simulink model "ForTest"  (R2023a)
settings: configuration reference "Reference" (kept outside this file)
libraries: trse_cmn_lib_V2 x2
settings Model: DataDictionary=For_common_config.sldd  Creator=C3020  LastModifiedBy=C9166
settings ConfigSetRef: SourceName=Reference

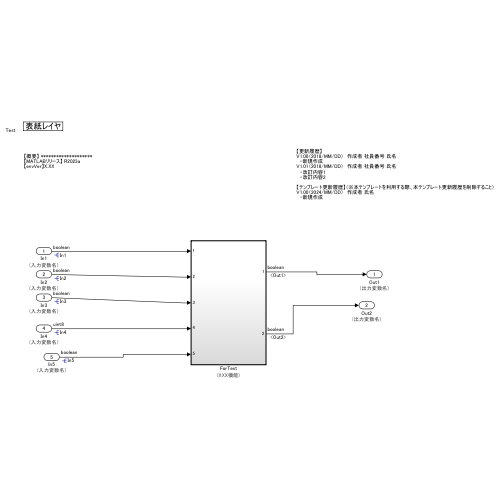
[thumbnail: Simulink's stored preview of the top-level diagram]
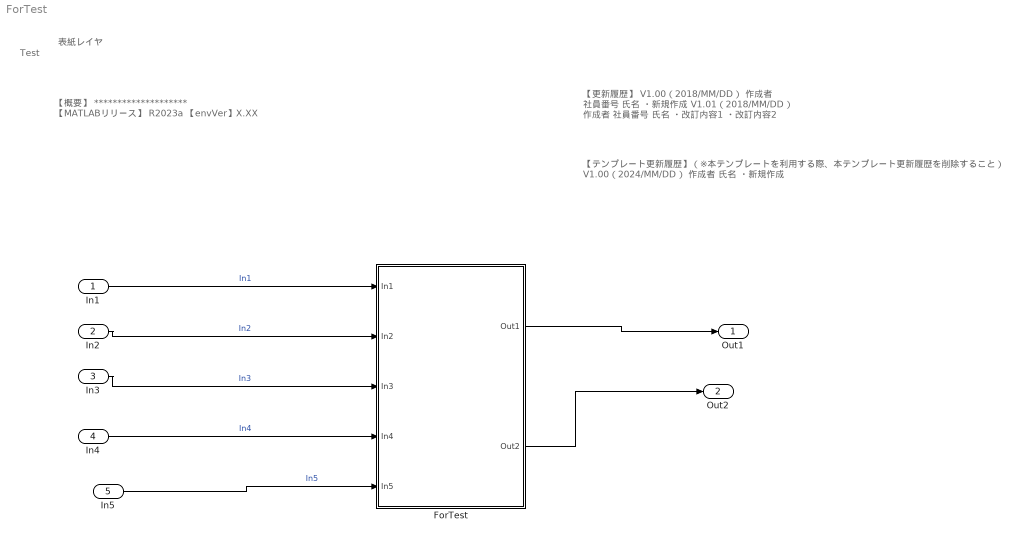
== system ForTest ==
  note: 表紙レイヤ
  note: 【更新履歴】
      | V1.00（2018/MM/DD）　作成者 社員番号 氏名
      | 　・新規作成
      | V1.01（2018/MM/DD）　作成者 社員番号 氏名
      | 　・改訂内容1
      | 　・改訂内容2
  note: 【テンプレート更新履歴】（※本テンプレートを利用する際、本テンプレート更新履歴を削除すること）
      | V1.00（2024/MM/DD）　作成者 氏名
      | 　・新規作成
  note: 【概要】 ********************
      | 【MATLABリリース】 R2023a
      | 【envVer】X.XX
  note: Test
  In1 : Inport  Description=入力変数名
      settings: AttributesFormatString=(%<Description>)
  In2 : Inport  Description=入力変数名  Port=2
      settings: AttributesFormatString=(%<Description>)
  In3 : Inport  Description=入力変数名  Port=3
      settings: AttributesFormatString=(%<Description>)
  In4 : Inport  Description=入力変数名  Port=4
      settings: AttributesFormatString=(%<Description>)
  In5 : Inport  Description=入力変数名  Port=5
      settings: AttributesFormatString=(%<Description>)
  ForTest : Subsystem  Description=XXX機能  TreatAsAtomicUnit=on
      settings: AttributesFormatString=(%<Description>)
  Out1 : Outport  Description=出力変数名
      settings: AttributesFormatString=(%<Description>)
  Out2 : Outport  Description=出力変数名  Port=2
      settings: AttributesFormatString=(%<Description>)
  wires:
  ForTest/1(Out1) -> Out1/1
  In1/1 -> ForTest/1(In1)  "In1"
  In2/1 -> ForTest/2(In2)  "In2"
  In3/1 -> ForTest/3(In3)  "In3"
  ForTest/2(Out2) -> Out2/1
  In4/1 -> ForTest/4(In4)  "In4"
  In5/1 -> ForTest/5(In5)  "In5"

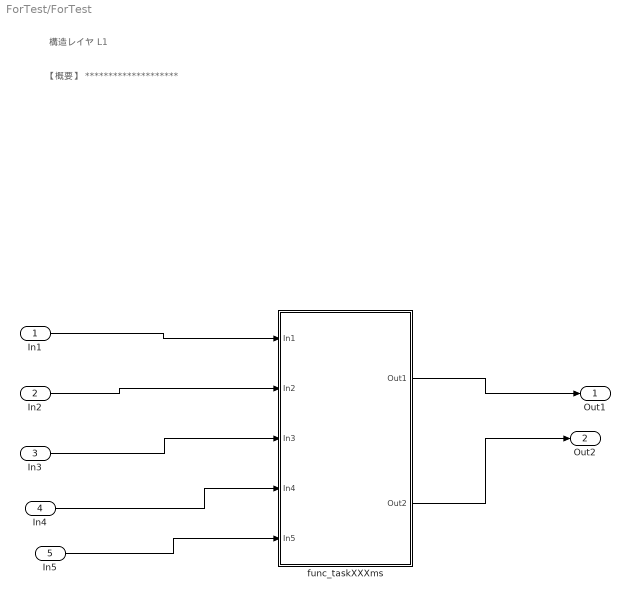
== system ForTest/ForTest ==
  note: 構造レイヤ L1
  note: 【概要】 ********************
  In1 : Inport  Description=入力変数名
      settings: AttributesFormatString=(%<Description>)
  In2 : Inport  Description=入力変数名  Port=2
      settings: AttributesFormatString=(%<Description>)
  In3 : Inport  Description=入力変数名  Port=3
      settings: AttributesFormatString=(%<Description>)
  In4 : Inport  Description=入力変数名  Port=4
      settings: AttributesFormatString=(%<Description>)
  In5 : Inport  Description=入力変数名  Port=5
      settings: AttributesFormatString=(%<Description>)
  func_taskXXXms : Subsystem  Description=XXX周期タスク  TreatAsAtomicUnit=on
      settings: AttributesFormatString=(%<Description>)
  Out1 : Outport  Description=出力変数名
      settings: AttributesFormatString=(%<Description>)
  Out2 : Outport  Description=出力変数名  Port=2
      settings: AttributesFormatString=(%<Description>)
  wires:
  func_taskXXXms/1(Out1) -> Out1/1
  In1/1 -> func_taskXXXms/1(In1)
  In2/1 -> func_taskXXXms/2(In2)
  In3/1 -> func_taskXXXms/3(In3)
  func_taskXXXms/2(Out2) -> Out2/1
  In4/1 -> func_taskXXXms/4(In4)
  In5/1 -> func_taskXXXms/5(In5)

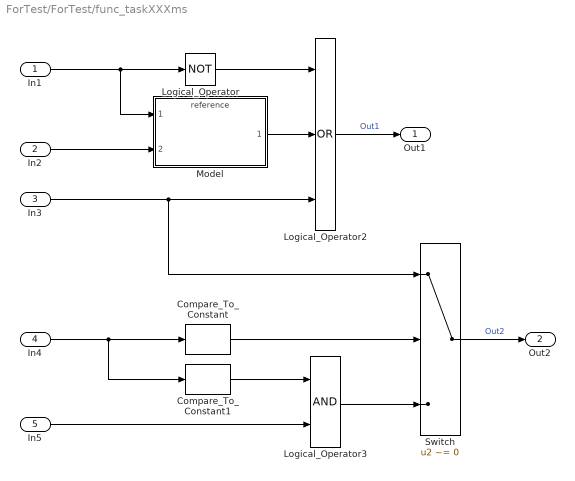
== system ForTest/ForTest/func_taskXXXms ==
  In1 : Inport  Description=入力変数名
      settings: AttributesFormatString=(%<Description>)
  In2 : Inport  Description=入力変数名  Port=2
      settings: AttributesFormatString=(%<Description>)
  In3 : Inport  Description=入力変数名  Port=3
      settings: AttributesFormatString=(%<Description>)
  In4 : Inport  Description=入力変数名  Port=4
      settings: AttributesFormatString=(%<Description>)
  In5 : Inport  Description=入力変数名  Port=5
      settings: AttributesFormatString=(%<Description>)
  Compare_To_Constant : trse_cmn_lib_V2/Logic and Bit Operations/Compare_To_Constant  Description=論理演算ライブラリ（定数比較）  relop=>=  const=3  InDataTypeStr=uint8  OutDataTypeStr=boolean
      settings: SourceProductName=TR Common Library V2
  Compare_To_Constant1 : trse_cmn_lib_V2/Logic and Bit Operations/Compare_To_Constant  Description=論理演算ライブラリ（定数比較）  relop=>=  const=6  InDataTypeStr=uint8  OutDataTypeStr=boolean
      settings: SourceProductName=TR Common Library V2
  Logical_Operator : Logic  Operator=NOT  OutDataTypeStr=boolean
  Logical_Operator2 : Logic  Operator=OR  Inputs=3  OutDataTypeStr=boolean
  Logical_Operator3 : Logic  OutDataTypeStr=boolean
  Model : ModelReference  Description=機能名  ModelNameDialog=reference.slx  SimulationMode=Normal  ModelReferenceVersion=1.56
      settings: AttributesFormatString=(%<Description>)
  Switch : Switch  Criteria=u2 ~= 0  RndMeth=Simplest
  Out1 : Outport  Description=出力変数名
      settings: AttributesFormatString=(%<Description>)
  Out2 : Outport  Description=出力変数名  Port=2
      settings: AttributesFormatString=(%<Description>)
  wires:
  In2/1 -> Model/2
  In1/1 -> Model/1, Logical_Operator/1
  In3/1 -> Switch/1, Logical_Operator2/3
  Logical_Operator/1 -> Logical_Operator2/1
  Logical_Operator2/1 -> Out1/1  "Out1"
  In4/1 -> Compare_To_Constant1/1, Compare_To_Constant/1
  Switch/1 -> Out2/1  "Out2"
  Compare_To_Constant/1 -> Switch/2
  In5/1 -> Logical_Operator3/2
  Model/1 -> Logical_Operator2/2
  Logical_Operator3/1 -> Switch/3
  Compare_To_Constant1/1 -> Logical_Operator3/1
